simulink model "Q2_2sim"  (R2016a)
settings: Solver=VariableStepAuto  StartTime=t_pend(N+1)  StopTime=max(t_pend)  MaxStep=0.01  RelTol=1e-3
values from neighbouring files (symbols this model uses):
  c = -M*l^2 * Theta(1)    [Q2_3.m]
  g = 9.81    [Q2_3.m]
  l = -g/Theta(2)    [Q2_3.m]
  M = 0.2    [Q2_3.m]
  N = 3    [Q2_2.m]    (also in Q2_3.m = 12; derivative_example.m)
undefined symbols (not defined in the file or in its folder): dtheta_pend, theta_pend
settings Model: Creator=masom  LastModifiedBy=masom

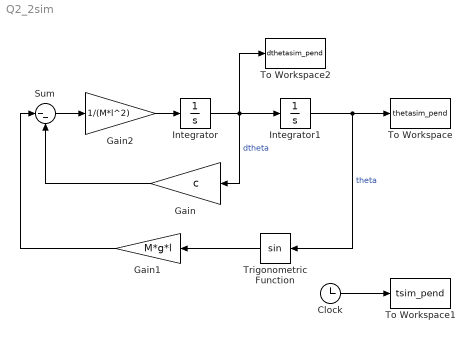
== system Q2_2sim ==
  Clock : Clock
  Gain : Gain  Gain=c
  Gain1 : Gain  Gain=M*g*l
  Gain2 : Gain  Gain=1/(M*l^2)
  Integrator : Integrator  InitialCondition=dtheta_pend(N+1)
  Integrator1 : Integrator  InitialCondition=theta_pend(N+1)
  Sum : Sum  Inputs=|--
  To Workspace : ToWorkspace  VariableName=thetasim_pend  SampleTime=-1
  To Workspace1 : ToWorkspace  VariableName=tsim_pend  SampleTime=-1
  To Workspace2 : ToWorkspace  VariableName=dthetasim_pend  SampleTime=-1
  Trigonometric Function : Trigonometry
  wires:
  Integrator/1 -> To Workspace2/1, Gain/1, Integrator1/1  "dtheta"
  Integrator1/1 -> Trigonometric Function/1, To Workspace/1  "theta"
  Sum/1 -> Gain2/1
  Gain/1 -> Sum/2
  Gain1/1 -> Sum/1
  Trigonometric Function/1 -> Gain1/1
  Clock/1 -> To Workspace1/1
  Gain2/1 -> Integrator/1
